simulink model "MSFartoystyring1_2"  (R2018a)
settings: Solver=ode45  StartTime=tstart  StopTime=tstop  RelTol=1e-3  EnableMultiTasking=on
values from neighbouring files (symbols this model uses):
  c = 0    [run.m]    (also in run_2.m = 1; run_task_1_4.m; run_task_1_6.m; run_task_1_6_new.m)
  kd = 0    [run.m]    (also in run_task_1_4.m; run_task_1_6.m; run_task_1_6_new.m = 2*zeta*omegan*(m+km)-d)
  kd_u = 0    [run.m]
  ki = omegan/10*kp    [run.m]    (also in run_task_1_4.m; run_task_1_6.m; run_task_1_6_new.m)
  ki_u = omegan/10*kp_u    [run.m]
  kp = (m+km)*omegan^2-k    [run.m]    (also in run_task_1_4.m; run_task_1_6.m; run_task_1_6_new.m)
  kp_u = (m+km)*omegan^2-k    [run.m]
  p0 = zeros(2,1)    [run.m]    (also in run_2.m = [1000 700]'; run_task_1_4.m; run_task_1_6.m; run_task_1_6_new.m)
  psi0 = 0    [run.m]    (also in run_2.m; run_task_1_4.m; run_task_1_6.m; run_task_1_6_new.m)
  r0 = 0    [run.m]    (also in run_2.m; run_task_1_4.m; run_task_1_6.m; run_task_1_6_new.m)
  tsamp = 10    [run.m]    (also in run_2.m; run_task_1_4.m; run_task_1_6.m; run_task_1_6_new.m)
  v0 = [3 0]'    [run.m]    (also in run_2.m = [6.63 0]'; run_task_1_4.m = [6.63 0]'; run_task_1_6.m = [0.001 0]'; run_task_1_6_new.m = [0.001 0]')
undefined symbols (not defined in the file or in its folder): msfartoystyring
settings Model: ExtModeAutoUpdateStatusClock=off  Creator=christh  LastModifiedBy=ada
settings DataIOCC: LimitDataPoints=on  SaveFormat=Array  SignalLoggingSaveFormat=ModelDataLogs
settings OptimizationCC: ExpressionDepthLimit=2147483647  InitFltsAndDblsToZero=on  LifeSpan=inf
settings DebuggingCC: UnderspecifiedInitializationDetection=Classic  MergeDetectMultiDrivingBlocksExec=none  SolverPrmCheckMsg=warning  FcnCallInpInsideContextMsg=warning  StateNameClashWarn=warning  SFUnexpectedBacktrackingDiag=warning  SFNoUnconditionalDefaultTransitionDiag=warning  SFExecutionAtInitializationDiag=none
settings HardwareCC: ProdBitPerPointer=32  ProdBitPerSizeT=32  ProdBitPerPtrDiffT=32  ProdLargestAtomicFloat=None  ProdIntDivRoundTo=Undefined  ProdEndianess=Unspecified  ProdWordSize=32  ProdHWDeviceType=32-bit Generic
settings ModelReferenceCC: PropagateSignalLabelsOutOfModel=off
settings CodeAppCC: StateflowObjectComments=on
settings GRTTargetCC: TargetLangStandard=C89/C90 (ANSI)  GeneratePreprocessorConditionals=Disable all  CombineOutputUpdateFcns=off  GRTInterface=on
settings ConfigComp: CovMetricSettings=dw  CovHtmlReporting=on  CovSaveCumulativeToWorkspaceVar=on  CovSaveSingleToWorkspaceVar=on  CovExternalEMLEnable=off

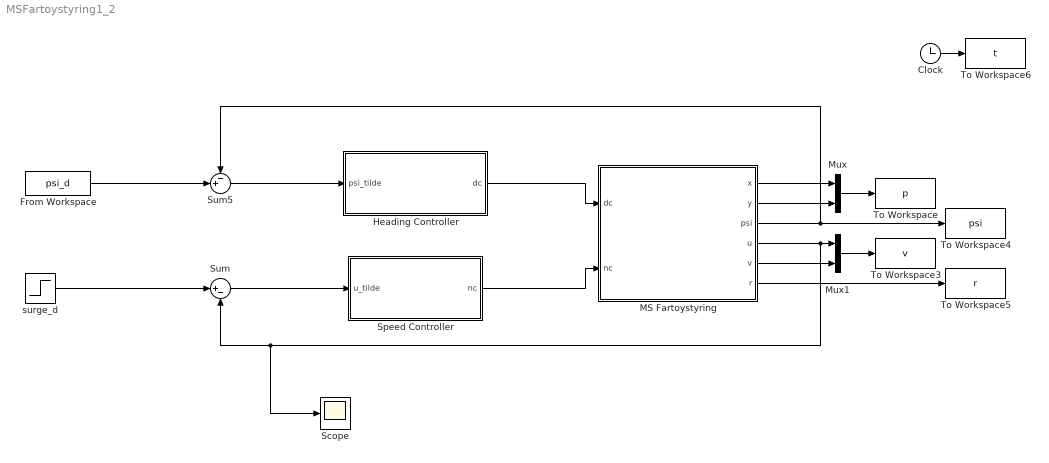
== system MSFartoystyring1_2 ==
  Clock : Clock
  From Workspace : FromWorkspace  VariableName=psi_d  SampleTime=0
  Heading Controller : Subsystem
  MS Fartoystyring : Subsystem  mask(MS Fartoystyring for Assignment 3 G&C){x0=p0(1), y0=p0(2), u0=v0(1), v0=v0(2), psi0=psi0, r0=r0, c=c}
      mask prompts: x0 "x(t0) (m)"; y0 "y(t0) (m)"; u0 "u(t0) (m/s)"; v0 "v(t0) (m/s)"; psi0 "psi(t0) (rad)"; r0 "r(t0) (rad/s)"; c "current (0 or 1)"
      mask help:
      | Block corresponding to Figure 1 in the assignment text. Gives the response of the ship.
      |
      | The design speed of MS Fartoystyring is u=8.23 m/s.
      |
      | Input:
      | dc: commanded rudder (rad), dmax=25*pi/180
      | nc: commanded shaft speed (rad/s), nmax=85*2*pi/60
      |
      | Output:
      | x: north pos (m)
      | y: east pos (m)
      | u: surge (m/s)
      | v: sway (m/s)
      | psi: heading (rad)
      | r: yaw (rad/s)
      mask Help: Comments, bugs and help requests can be directed to the TA. Email on course website.
  Mux : Mux  Inputs=2
  Mux1 : Mux  Inputs=2
  Scope : Scope
  Speed Controller : Subsystem
  Sum : Sum  Inputs=|+-
  Sum5 : Sum  Inputs=-+|
  To Workspace : ToWorkspace  VariableName=p  SampleTime=tsamp
  To Workspace3 : ToWorkspace  VariableName=v  SampleTime=tsamp
  To Workspace4 : ToWorkspace  VariableName=psi  SampleTime=tsamp
  To Workspace5 : ToWorkspace  VariableName=r  SampleTime=tsamp
  To Workspace6 : ToWorkspace  VariableName=t  SampleTime=tsamp
  surge_d : Step  Time=1250  Before=3  After=7  SampleTime=0
  wires:
  Clock/1 -> To Workspace6/1
  MS Fartoystyring/1(x) -> Mux/1
  MS Fartoystyring/2(y) -> Mux/2
  MS Fartoystyring/5(v) -> Mux1/2
  Mux/1 -> To Workspace/1
  Mux1/1 -> To Workspace3/1
  MS Fartoystyring/3(psi) -> Sum5/1, To Workspace4/1
  MS Fartoystyring/6(r) -> To Workspace5/1
  surge_d/1 -> Sum/1
  MS Fartoystyring/4(u) -> Scope/1, Sum/2, Mux1/1
  From Workspace/1 -> Sum5/2
  Sum5/1 -> Heading Controller/1(psi_tilde)
  Heading Controller/1(dc) -> MS Fartoystyring/1(dc)
  Sum/1 -> Speed Controller/1(u_tilde)
  Speed Controller/1(nc) -> MS Fartoystyring/2(nc)

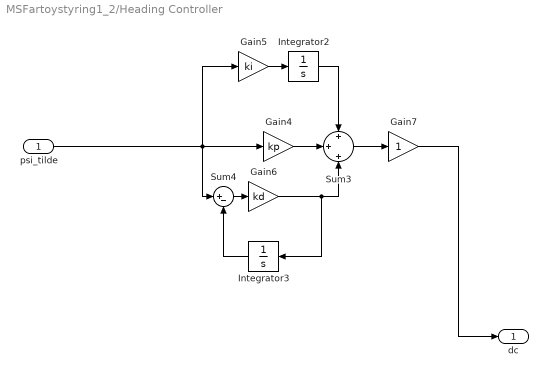
== system MSFartoystyring1_2/Heading Controller ==
  psi_tilde : Inport
  Gain4 : Gain  Gain=kp
  Gain5 : Gain  Gain=ki
  Gain6 : Gain  Gain=kd
  Gain7 : Gain
  Integrator2 : Integrator
  Integrator3 : Integrator
  Sum3 : Sum  Inputs=+|+|+
  Sum4 : Sum  Inputs=|+-
  dc : Outport
  wires:
  Gain4/1 -> Sum3/2
  Integrator3/1 -> Sum4/2
  Gain5/1 -> Integrator2/1
  Gain7/1 -> dc/1
  psi_tilde/1 -> Sum4/1, Gain4/1, Gain5/1
  Sum3/1 -> Gain7/1
  Sum4/1 -> Gain6/1
  Integrator2/1 -> Sum3/1
  Gain6/1 -> Integrator3/1, Sum3/3

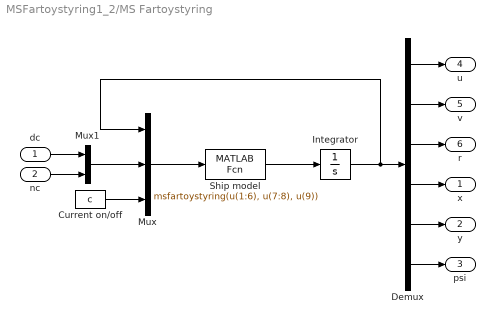
== system MSFartoystyring1_2/MS Fartoystyring ==
  dc : Inport
  nc : Inport  Port=2
  Current on/off : Constant  Value=c
  Demux : Demux  Outputs=6
  Integrator : Integrator  InitialCondition=[u0 v0 r0 x0 y0 psi0]'
  Mux : Mux  Inputs=3
  Mux1 : Mux  Inputs=2
  Ship model : MATLABFcn  MATLABFcn=msfartoystyring(u(1:6), u(7:8), u(9))  OutputDimensions=6
  x : Outport
  y : Outport  Port=2
  psi : Outport  Port=3
  u : Outport  Port=4
  v : Outport  Port=5
  r : Outport  Port=6
  wires:
  Integrator/1 -> Mux/1, Demux/1
  Mux1/1 -> Mux/2
  dc/1 -> Mux1/1
  nc/1 -> Mux1/2
  Demux/1 -> u/1
  Demux/2 -> v/1
  Demux/3 -> r/1
  Demux/4 -> x/1
  Demux/5 -> y/1
  Demux/6 -> psi/1
  Current on/off/1 -> Mux/3
  Ship model/1 -> Integrator/1
  Mux/1 -> Ship model/1

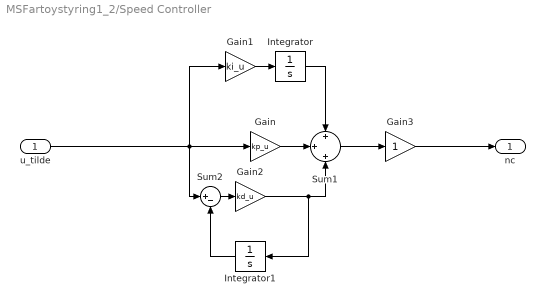
== system MSFartoystyring1_2/Speed Controller ==
  u_tilde : Inport
  Gain : Gain  Gain=kp_u
  Gain1 : Gain  Gain=ki_u
  Gain2 : Gain  Gain=kd_u
  Gain3 : Gain
  Integrator : Integrator
  Integrator1 : Integrator
  Sum1 : Sum  Inputs=+|+|+
  Sum2 : Sum  Inputs=|+-
  nc : Outport
  wires:
  Gain2/1 -> Integrator1/1, Sum1/3
  u_tilde/1 -> Sum2/1, Gain/1, Gain1/1
  Gain/1 -> Sum1/2
  Sum1/1 -> Gain3/1
  Gain1/1 -> Integrator/1
  Integrator/1 -> Sum1/1
  Gain3/1 -> nc/1
  Sum2/1 -> Gain2/1
  Integrator1/1 -> Sum2/2
